simulink model "PID_model"  (R2021a)
settings: Solver=VariableStepAuto  StartTime=0.0  StopTime=35  RelTol=1e-3
values from neighbouring files (symbols this model uses):
  Kd = 2    [PID_model_script.m]
  Ki = 2.5    [PID_model_script.m]
  Kp = 5    [PID_model_script.m]
  Kpert = 0.1    [PID_model_script.m]
  Kproc = 1    [PID_model_script.m]
  N = 1    [PID_model_script.m]
  Pert = 15000    [PID_model_script.m]
  SP = 5000    [PID_model_script.m]
  Tau = 0.5    [PID_model_script.m]
settings Model: Creator=javie  LastModifiedBy=javie

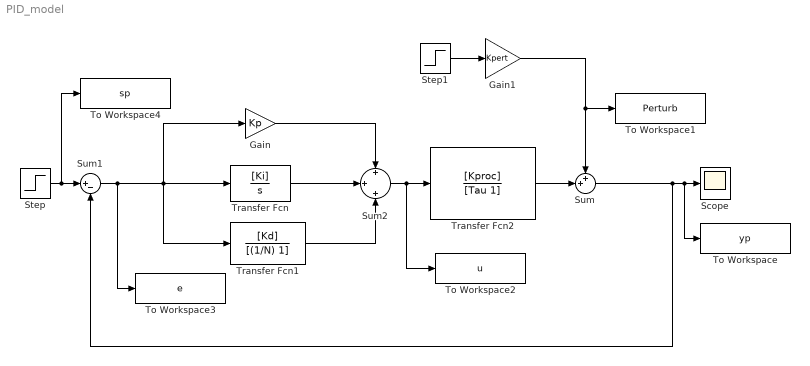
== system PID_model ==
  Gain : Gain  Gain=Kp
  Gain1 : Gain  Gain=Kpert
  Scope : Scope
  Step : Step  After=SP  SampleTime=0
  Step1 : Step  Time=20  After=Pert  SampleTime=0
  Sum : Sum  Inputs=++|
  Sum1 : Sum  Inputs=|+-
  Sum2 : Sum  Inputs=+|+|+
  To Workspace : ToWorkspace  VariableName=yp  SaveFormat=Timeseries  SampleTime=-1
  To Workspace1 : ToWorkspace  VariableName=Perturb  SaveFormat=Timeseries  SampleTime=-1
  To Workspace2 : ToWorkspace  VariableName=u  SaveFormat=Timeseries  SampleTime=-1
  To Workspace3 : ToWorkspace  VariableName=e  SaveFormat=Timeseries  SampleTime=-1
  To Workspace4 : ToWorkspace  VariableName=sp  SaveFormat=Timeseries  SampleTime=-1
  Transfer Fcn : TransferFcn  Numerator=[Ki]  Denominator=[1 0]
  Transfer Fcn1 : TransferFcn  Numerator=[Kd]  Denominator=[(1/N) 1]
  Transfer Fcn2 : TransferFcn  Numerator=[Kproc]  Denominator=[Tau 1]
  wires:
  Sum/1 -> Sum1/2, To Workspace/1, Scope/1
  Step1/1 -> Gain1/1
  Sum2/1 -> To Workspace2/1, Transfer Fcn2/1
  Transfer Fcn2/1 -> Sum/2
  Gain1/1 -> To Workspace1/1, Sum/1
  Gain/1 -> Sum2/1
  Transfer Fcn/1 -> Sum2/2
  Transfer Fcn1/1 -> Sum2/3
  Step/1 -> To Workspace4/1, Sum1/1
  Sum1/1 -> To Workspace3/1, Transfer Fcn1/1, Gain/1, Transfer Fcn/1
